simulink model "LQRControl"  (R2022a)
settings: Solver=VariableStepAuto  StartTime=0.0  StopTime=60  RelTol=1e-3
undefined symbols (not defined in the file): A2, Ao, B2, Bo, C2, C2a, Co, delay, den, Do, Go, Ho, Kdlqr, Kdlqr2, Klqr, Klqr2, num, T
libraries: simulink x5
settings Model: Creator=donovan  LastModifiedBy=donovan

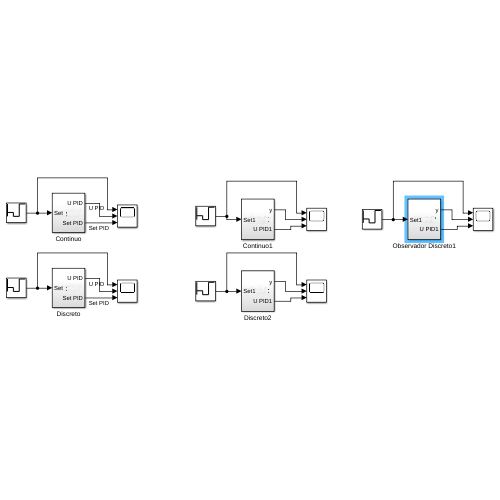
[thumbnail: Simulink's stored preview of the top-level diagram]
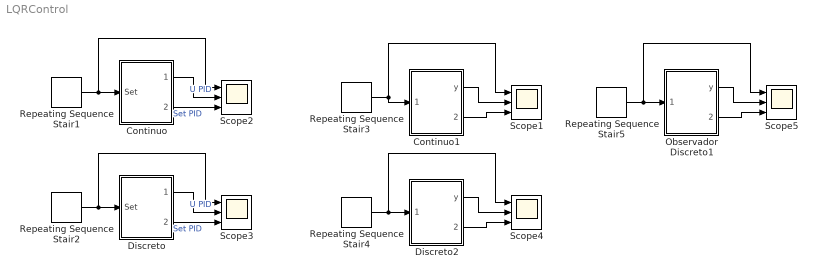
== system LQRControl ==
  Continuo : Subsystem
  Continuo1 : Subsystem
  Discreto : Subsystem
  Discreto2 : Subsystem
  Observador Discreto1 : Subsystem
  Repeating Sequence Stair{1..5} (5 alike) : simulink/Sources/Repeating Sequence Stair  OutValues=[60 10 180].'  tsamp=10  OutMin=[]  OutMax=[]  OutDataTypeStr=double  OutputDataTypeScalingMode=double  OutDataType=fixdt(0,8)  ConRadixGroup=Best Precision: Vector-wise  OutScaling=2^-12
  Scope{1..5} (5 alike) : Scope  NumInputPorts=3
  wires:
  Discreto/1(U PID) -> Scope3/2  "U PID"
  Discreto/2(Set PID) -> Scope3/3  "Set PID"
  Repeating Sequence Stair2/1 -> Scope3/1, Discreto/1(Set)
  Continuo/2(Set PID) -> Scope2/3  "Set PID"
  Repeating Sequence Stair1/1 -> Scope2/1, Continuo/1(Set)
  Continuo/1(U PID) -> Scope2/2  "U PID"
  Repeating Sequence Stair3/1 -> Scope1/1, Continuo1/1(Set1)
  Continuo1/1(y) -> Scope1/2
  Continuo1/2(U PID1) -> Scope1/3
  Repeating Sequence Stair4/1 -> Scope4/1, Discreto2/1(Set1)
  Discreto2/2(U PID1) -> Scope4/3
  Discreto2/1(y) -> Scope4/2
  Repeating Sequence Stair5/1 -> Scope5/1, Observador Discreto1/1(Set1)
  Observador Discreto1/1(y) -> Scope5/2
  Observador Discreto1/2(U PID1) -> Scope5/3

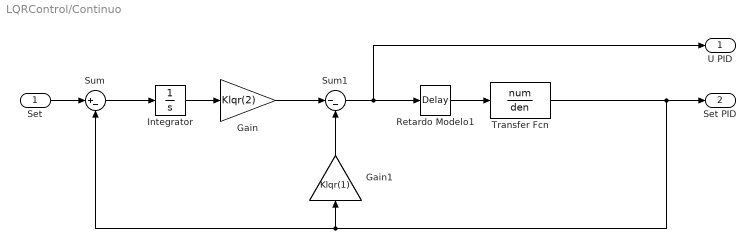
== system LQRControl/Continuo ==
  Set : Inport
  Gain : Gain  Gain=Klqr(2)
  Gain1 : Gain  Gain=Klqr(1)
  Integrator : Integrator
  Retardo Modelo1 : TransportDelay  DelayTime=delay
  Sum : Sum  Inputs=|+-
  Sum1 : Sum  Inputs=|--
  Transfer Fcn : TransferFcn  Numerator=num  Denominator=den
  U PID : Outport
  Set PID : Outport  Port=2
  wires:
  Transfer Fcn/1 -> Set PID/1, Gain1/1, Sum/2
  Retardo Modelo1/1 -> Transfer Fcn/1
  Set/1 -> Sum/1
  Sum/1 -> Integrator/1
  Integrator/1 -> Gain/1
  Sum1/1 -> U PID/1, Retardo Modelo1/1
  Gain/1 -> Sum1/1
  Gain1/1 -> Sum1/2

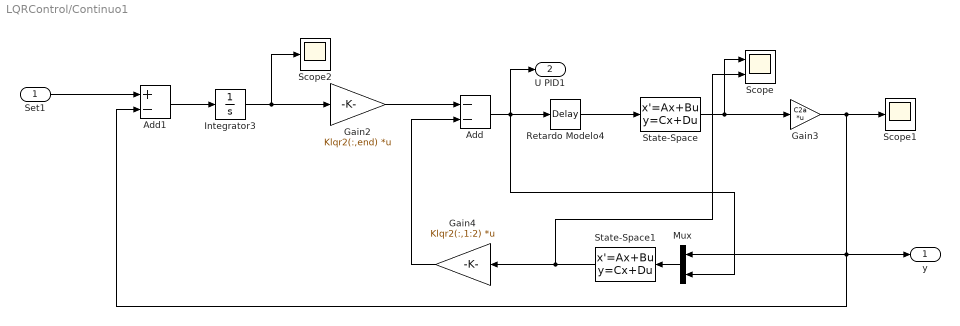
== system LQRControl/Continuo1 ==
  Set1 : Inport
  Add : Sum  Inputs=--
  Add1 : Sum  Inputs=+-
  Gain2 : Gain  Gain=Klqr2(:,end)  Multiplication=Matrix(K*u)
  Gain3 : Gain  Gain=C2a  Multiplication=Matrix(K*u)
  Gain4 : Gain  Gain=Klqr2(:,1:2)  Multiplication=Matrix(K*u)
  Integrator3 : Integrator
  Mux : Mux  Inputs=2
  Retardo Modelo4 : TransportDelay  DelayTime=delay
  Scope : Scope  NumInputPorts=2
  Scope1 : Scope
  Scope2 : Scope
  State-Space : StateSpace  A=A2  B=B2  C=C2  D=zeros(2,2)  InitialCondition=0
  State-Space1 : StateSpace  A=Ao  B=Bo  C=Co  D=Do  InitialCondition=0  AllowTunableDMatrix=on
  y : Outport
  U PID1 : Outport  Port=2
  wires:
  State-Space/1 -> Gain3/1, Scope/1
  Gain4/1 -> Add/2
  Add1/1 -> Integrator3/1
  Integrator3/1 -> Scope2/1, Gain2/1
  Gain2/1 -> Add/1
  Retardo Modelo4/1 -> State-Space/1
  Add/1 -> Mux/2, U PID1/1, Retardo Modelo4/1
  Set1/1 -> Add1/1
  Gain3/1 -> Mux/1, y/1, Add1/2, Scope1/1
  State-Space1/1 -> Scope/2, Gain4/1
  Mux/1 -> State-Space1/1

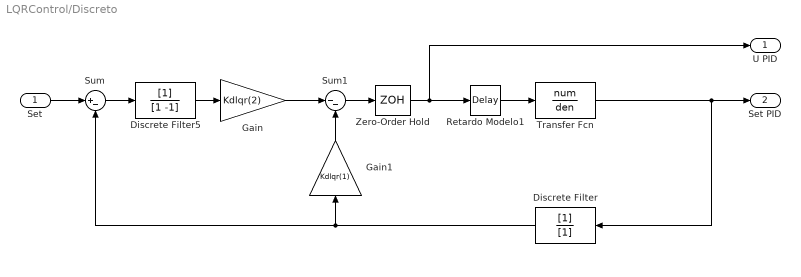
== system LQRControl/Discreto ==
  Set : Inport
  Discrete Filter : DiscreteFilter  Denominator=[1]  SampleTime=T
  Discrete Filter5 : DiscreteFilter  Denominator=[1 -1]  SampleTime=T
  Gain : Gain  Gain=Kdlqr(2)
  Gain1 : Gain  Gain=Kdlqr(1)
  Retardo Modelo1 : TransportDelay  DelayTime=delay
  Sum : Sum  Inputs=|+-
  Sum1 : Sum  Inputs=|--
  Transfer Fcn : TransferFcn  Numerator=num  Denominator=den
  Zero-Order Hold : ZeroOrderHold  SampleTime=T
  U PID : Outport
  Set PID : Outport  Port=2
  wires:
  Transfer Fcn/1 -> Set PID/1, Discrete Filter/1
  Retardo Modelo1/1 -> Transfer Fcn/1
  Set/1 -> Sum/1
  Sum/1 -> Discrete Filter5/1
  Discrete Filter5/1 -> Gain/1
  Sum1/1 -> Zero-Order Hold/1
  Gain/1 -> Sum1/1
  Gain1/1 -> Sum1/2
  Discrete Filter/1 -> Sum/2, Gain1/1
  Zero-Order Hold/1 -> U PID/1, Retardo Modelo1/1

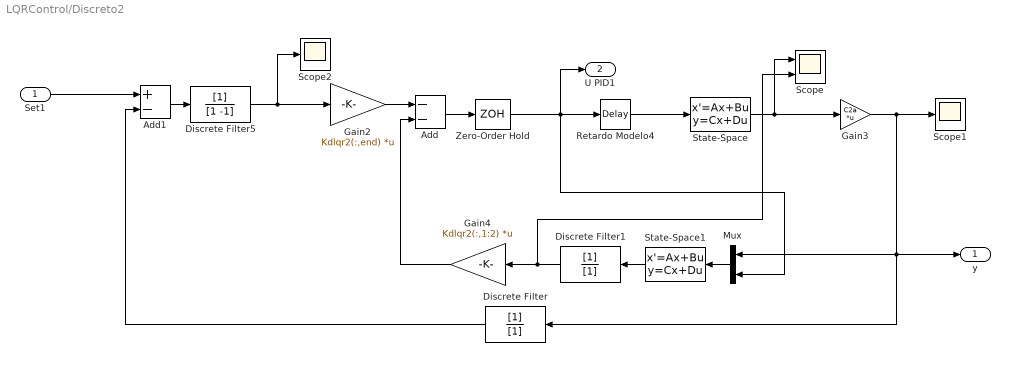
== system LQRControl/Discreto2 ==
  Set1 : Inport
  Add : Sum  Inputs=--
  Add1 : Sum  Inputs=+-
  Discrete Filter : DiscreteFilter  Denominator=[1]  SampleTime=T
  Discrete Filter1 : DiscreteFilter  Denominator=[1]  SampleTime=T
  Discrete Filter5 : DiscreteFilter  Denominator=[1 -1]  SampleTime=T
  Gain2 : Gain  Gain=Kdlqr2(:,end)  Multiplication=Matrix(K*u)
  Gain3 : Gain  Gain=C2a  Multiplication=Matrix(K*u)
  Gain4 : Gain  Gain=Kdlqr2(:,1:2)  Multiplication=Matrix(K*u)
  Mux : Mux  Inputs=2
  Retardo Modelo4 : TransportDelay  DelayTime=delay
  Scope : Scope  NumInputPorts=2
  Scope1 : Scope
  Scope2 : Scope
  State-Space : StateSpace  A=A2  B=B2  C=C2  D=zeros(2,2)  InitialCondition=0
  State-Space1 : StateSpace  A=Ao  B=Bo  C=Co  D=Do  InitialCondition=0  AllowTunableDMatrix=on
  Zero-Order Hold : ZeroOrderHold  SampleTime=T
  y : Outport
  U PID1 : Outport  Port=2
  wires:
  State-Space/1 -> Gain3/1, Scope/1
  Gain4/1 -> Add/2
  Add1/1 -> Discrete Filter5/1
  Discrete Filter5/1 -> Scope2/1, Gain2/1
  Gain2/1 -> Add/1
  Retardo Modelo4/1 -> State-Space/1
  Add/1 -> Zero-Order Hold/1
  Set1/1 -> Add1/1
  Gain3/1 -> Mux/1, y/1, Discrete Filter/1, Scope1/1
  State-Space1/1 -> Discrete Filter1/1
  Mux/1 -> State-Space1/1
  Discrete Filter/1 -> Add1/2
  Discrete Filter1/1 -> Scope/2, Gain4/1
  Zero-Order Hold/1 -> Mux/2, U PID1/1, Retardo Modelo4/1

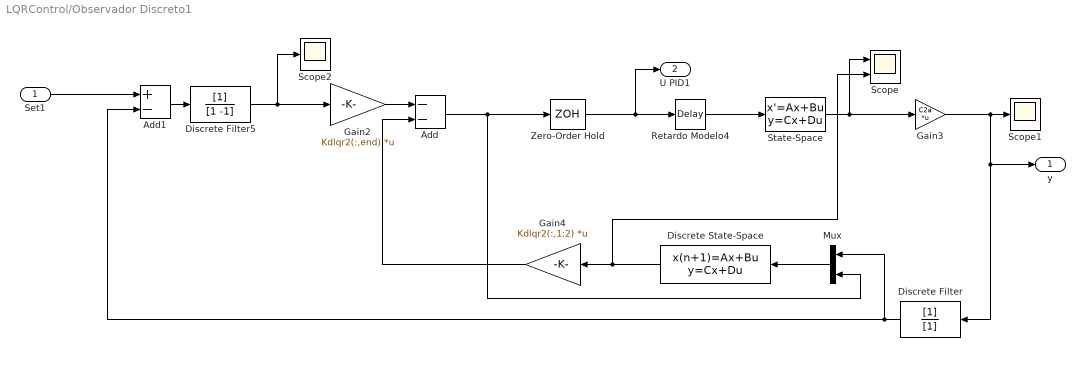
== system LQRControl/Observador Discreto1 ==
  Set1 : Inport
  Add : Sum  Inputs=--
  Add1 : Sum  Inputs=+-
  Discrete Filter : DiscreteFilter  Denominator=[1]  SampleTime=T
  Discrete Filter5 : DiscreteFilter  Denominator=[1 -1]  SampleTime=T
  Discrete State-Space : DiscreteStateSpace  A=Go  B=Ho  C=Co  D=Do  SampleTime=T
  Gain2 : Gain  Gain=Kdlqr2(:,end)  Multiplication=Matrix(K*u)
  Gain3 : Gain  Gain=C2a  Multiplication=Matrix(K*u)
  Gain4 : Gain  Gain=Kdlqr2(:,1:2)  Multiplication=Matrix(K*u)
  Mux : Mux  Inputs=2
  Retardo Modelo4 : TransportDelay  DelayTime=delay
  Scope : Scope  NumInputPorts=2
  Scope1 : Scope
  Scope2 : Scope
  State-Space : StateSpace  A=A2  B=B2  C=C2  D=zeros(2,2)  InitialCondition=0
  Zero-Order Hold : ZeroOrderHold  SampleTime=T
  y : Outport
  U PID1 : Outport  Port=2
  wires:
  State-Space/1 -> Gain3/1, Scope/1
  Gain4/1 -> Add/2
  Add1/1 -> Discrete Filter5/1
  Discrete Filter5/1 -> Scope2/1, Gain2/1
  Gain2/1 -> Add/1
  Retardo Modelo4/1 -> State-Space/1
  Add/1 -> Zero-Order Hold/1, Mux/2
  Set1/1 -> Add1/1
  Gain3/1 -> y/1, Discrete Filter/1, Scope1/1
  Mux/1 -> Discrete State-Space/1
  Discrete State-Space/1 -> Scope/2, Gain4/1
  Zero-Order Hold/1 -> U PID1/1, Retardo Modelo4/1
  Discrete Filter/1 -> Mux/1, Add1/2
